simulink model "test_bu01_2018b_tuning"  (R2018b)
settings: Solver=FixedStepAuto  StartTime=0.0  StopTime=10  FixedStep=0.001  RelTol=1e-3
model workspace (MAT data in the model file):
  B1 = 0.0229925610147
  B2 = -0.371283802987
  B3 = -0.920624315565
  B4 = -0.0418343375444
  B5 = -0.493210333206
  B6 = 0
  B7 = -0.0892006103314
  B8 = -0.433620647544
  Ixx = 0.8
  Iyy = 2.075
  Izz = 1.25
  K = 0.92
  K1 = 0.96
  M1 = [1 1 -1 0.151123095698]
  M2 = [1 0 1 0.728919165533]
  M3 = [-1 0 -1 0]
  M4 = [-1 1 1 0.279370204784]
  M5 = [0 -1 0 0.953177368176]
  M6 = [0 -1 0 -1]
  M7 = [0 -1 0 0.164756597211]
  M8 = [0 -1 0 0.72330475505]
  Mass = 11.5
  b = 0
libraries: simulink x4, vrlib x4, shared6dof x1
(part 1 of 3)
settings Model: Creator=Administrator  LastModifiedBy=39926
settings DataIOCC: ReturnWorkspaceOutputs=on

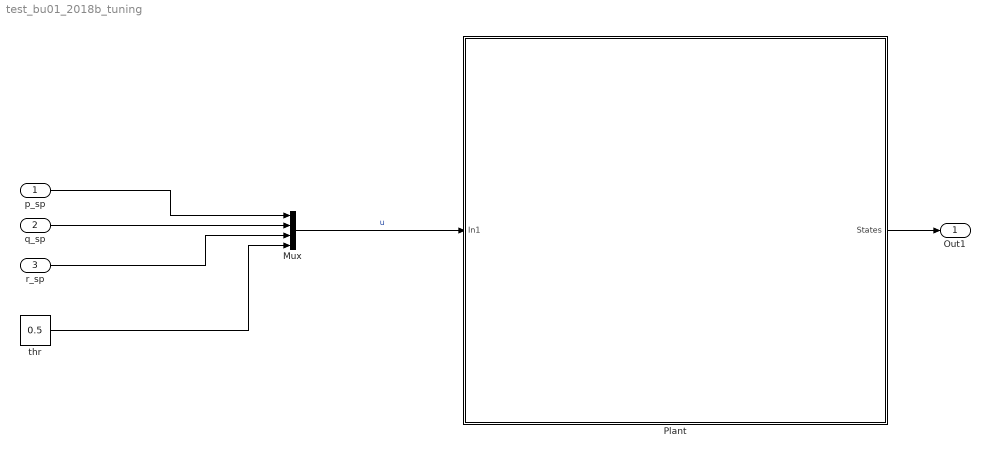
== system test_bu01_2018b_tuning ==
  "p_sp " : Inport
  q_sp : Inport  Port=2
  "r_sp " : Inport  Port=3
  Mux : Mux
  Plant : Subsystem
      mask Display: image('airframe.jpg');
  thr : Constant  Value=0.5
  Out1 : Outport
  wires:
  Mux/1 -> Plant/1(In1)  "u"
  q_sp/1 -> Mux/2
  "r_sp "/1 -> Mux/3
  Plant/1(States) -> Out1/1
  thr/1 -> Mux/4
  "p_sp "/1 -> Mux/1

== system test_bu01_2018b_tuning/Plant ==
  In1 : Inport
  Demux{,1..3} (4 alike) : Demux  Outputs=3
  Terminator{,3,5..9} (7 alike) : Terminator
  bu01_model : Subsystem  mask{Density=1.185}
      mask prompts: Density "空气密度D"
  混控器 : Subsystem
  Out Bus Element : Outport  PortName=States  Element=Xe
  Out Bus Element1 : Outport  PortName=States  Element=Ye
  Out Bus Element2 : Outport  PortName=States  Element=Ze
  Out Bus Element3 : Outport  PortName=States  Element=phi
  Out Bus Element4 : Outport  PortName=States  Element=theta
  Out Bus Element5 : Outport  PortName=States  Element=psi
  Out Bus Element6 : Outport  PortName=States  Element=u
  Out Bus Element7 : Outport  PortName=States  Element=v
  Out Bus Element8 : Outport  PortName=States  Element=w
  Out Bus Element9 : Outport  PortName=States  Element=p
  Out Bus Element10 : Outport  PortName=States  Element=q
  Out Bus Element11 : Outport  PortName=States  Element=r
  wires:
  混控器/1(PWM) -> bu01_model/1(PWM)
  bu01_model/6(Wb) -> Demux3/1
  bu01_model/7(dw/dt) -> Terminator5/1
  In1/1 -> 混控器/1(CtrlIn)
  bu01_model/1(Ve) -> Terminator/1
  bu01_model/3(ang) -> Demux1/1
  bu01_model/2(Xe) -> Demux/1
  bu01_model/4(DCM_e2b) -> Terminator3/1
  bu01_model/5(Vb) -> Demux2/1
  bu01_model/8(Abb) -> Terminator6/1
  bu01_model/9(T) -> Terminator7/1
  bu01_model/10(M) -> Terminator8/1
  bu01_model/11(Abe) -> Terminator9/1
  Demux/1 -> Out Bus Element/1
  Demux/2 -> Out Bus Element1/1
  Demux/3 -> Out Bus Element2/1
  Demux1/1 -> Out Bus Element3/1
  Demux1/2 -> Out Bus Element4/1
  Demux1/3 -> Out Bus Element5/1
  Demux2/1 -> Out Bus Element6/1
  Demux2/2 -> Out Bus Element7/1
  Demux2/3 -> Out Bus Element8/1
  Demux3/2 -> Out Bus Element10/1
  Demux3/1 -> Out Bus Element9/1
  Demux3/3 -> Out Bus Element11/1

== system test_bu01_2018b_tuning/Plant/bu01_model ==
  PWM : Inport
  6DOF (Quaternion) : shared6dof/6DOF (Euler Angles)  units=Metric (MKS)  mtype=Fixed  rep=Quaternion  xme_0=[0 0 0]  Vm_0=[0 0 0]  eul_0=[0 0 0]  pm_0=[0 0 0]  mass_0=Mass  mass_e=0.5  mass_f=2.0  inertia=[Ixx 0 0; 0 Iyy 0;0 0 Izz]  inertia_e=eye(3)  inertia_f=2*eye(3)  k_quat=1.0  vre_flag=on  abi_flag=on  aMode=0  xme_statename=''  Vm_statename=''  eul_statename=''  quat_statename=''  pm_statename=''  mass_statename=''
      settings: SourceProductBaseCode=AE
  Add : Sum  Inputs=3
  Add1 : Sum
  Constant : Constant  Value=Density
  Constant1 : Constant  Value=[0 0 0]
  Constant2 : Constant  Value=[0 0 0]
  PWM2Um : Subsystem
  动力系统模型 : Subsystem
  空气动力模型 : ModelReference  ModelNameDialog=BU01AM.slx  SimulationMode=Normal  ModelReferenceVersion=1.55
  重力模型 : Subsystem  mask{G=9.81, m=11.5}
      mask prompts: G "重力加速度G"; m "质量m"
  Ve : Outport
  Xe : Outport  Port=2
  ang : Outport  Port=3
  DCM_e2b : Outport  Port=4
  Vb : Outport  Port=5
  Wb : Outport  Port=6
  dw/dt : Outport  Port=7
  Abb : Outport  Port=8
  T : Outport  Port=9
  M : Outport  Port=10
  Abe : Outport  Port=11
  wires:
  Add1/1 -> M/1, 6DOF (Quaternion)/2  "M"
  6DOF (Quaternion)/1 -> Ve/1
  6DOF (Quaternion)/3 -> ang/1
  6DOF (Quaternion)/2 -> Xe/1
  6DOF (Quaternion)/4 -> 重力模型/1(DCM_e2b), DCM_e2b/1
  Add/1 -> T/1, 6DOF (Quaternion)/1  "T"
  6DOF (Quaternion)/7 -> dw/dt/1
  6DOF (Quaternion)/8 -> Abb/1
  6DOF (Quaternion)/5 -> Vb/1
  6DOF (Quaternion)/6 -> 空气动力模型/2, Wb/1
  6DOF (Quaternion)/9 -> Abe/1
  Constant/1 -> 空气动力模型/4
  重力模型/1(Fb_mg) -> Add/1  "mg_F"
  动力系统模型/1(Fb) -> Add/2  "Mot_F"
  空气动力模型/1 -> Add/3  "AM_F"
  空气动力模型/2 -> Add1/2  "AM_M"
  动力系统模型/2(Mb) -> Add1/1  "Mot_M"
  Constant1/1 -> 空气动力模型/3, 动力系统模型/3(Wb)
  Constant2/1 -> 空气动力模型/1, 动力系统模型/2(Vb)
  PWM/1 -> PWM2Um/1(PWM)
  PWM2Um/1(Um) -> 动力系统模型/1("Um ")

== system test_bu01_2018b_tuning/Plant/混控器 ==
  note: 机体构型描述：
      |           ^
      |           ||
      | 1P   -  ||  -   4N
      | 2N   -  ||  -   3P
      |            ||
      |            ||
      | -------------------
      | 5N  6N   7N 8N
  CtrlIn : Inport
  Bias{1..4} (4 alike) : Bias  Bias=[0 b 0 b]
  Demux : Demux  Outputs=8
  Gain : Gain  Gain="[1 1  -1 1]"
  Gain1 : Gain  Gain="[1 0  1 1]"
  Gain10 : Gain  Gain=K1
  Gain11 : Gain  Gain=K
  Gain2 : Gain  Gain=[-1 0 -1 1]
  Gain3 : Gain  Gain=[-1 1 1 1]
  Gain{4..6,8} (4 alike) : Gain  Gain=[0 -1 0 1]
  Gain7 : Gain  Gain=K
  Gain9 : Gain  Gain=K1
  Mux : Mux  Inputs=8
  Saturation : Saturate  UpperLimit=1  LowerLimit=0
  Scope : Scope
  Scope1 : Scope  NumInputPorts=8
  Sum of Elements{,1..7} (8 alike) : Sum  Inputs=+
  PWM : Outport
  wires:
  Sum of Elements/1 -> Mux/1
  Gain/1 -> Sum of Elements/1
  Gain2/1 -> Sum of Elements2/1
  Gain3/1 -> Sum of Elements3/1
  CtrlIn/1 -> Scope/1, Gain3/1, Gain4/1, Gain5/1, Gain8/1, Gain6/1, Gain1/1, Gain/1, Gain2/1
  Gain1/1 -> Sum of Elements1/1
  Bias3/1 -> Sum of Elements7/1
  Saturation/1 -> PWM/1, Demux/1
  Sum of Elements1/1 -> Mux/2
  Sum of Elements2/1 -> Mux/3
  Sum of Elements3/1 -> Mux/4
  Sum of Elements4/1 -> Mux/5
  Sum of Elements5/1 -> Mux/6
  Sum of Elements6/1 -> Mux/7
  Sum of Elements7/1 -> Mux/8
  Demux/1 -> Scope1/1  "m1"
  Demux/2 -> Scope1/2  "m2"
  Demux/3 -> Scope1/3  "m3"
  Demux/4 -> Scope1/4  "m4"
  Demux/5 -> Scope1/5  "m5"
  Demux/6 -> Scope1/6  "m6"
  Demux/7 -> Scope1/7  "m7"
  Demux/8 -> Scope1/8  "m8"
  Gain7/1 -> Bias3/1
  Gain8/1 -> Gain7/1
  Bias1/1 -> Sum of Elements6/1
  Gain6/1 -> Gain9/1
  Gain9/1 -> Bias1/1
  Bias2/1 -> Sum of Elements5/1
  Gain5/1 -> Gain10/1
  Gain10/1 -> Bias2/1
  Bias4/1 -> Sum of Elements4/1
  Gain4/1 -> Gain11/1
  Gain11/1 -> Bias4/1
  Mux/1 -> Saturation/1

== system test_bu01_2018b_tuning/Plant/bu01_model/PWM2Um ==
  PWM : Inport
  120AESC : Subsystem
  40AESC : Subsystem
  Constant2 : Constant  Value=25.2
  Demux : Demux  Outputs=2
  Demux1 : Demux  Outputs=8
  Mux : Mux  Inputs=2
  Saturation : Saturate  UpperLimit=1  LowerLimit=0
  Scope : Scope  NumInputPorts=8
  Um : Outport
  wires:
  Saturation/1 -> Demux/1
  PWM/1 -> Saturation/1
  120AESC/1(Out1) -> Mux/2
  Mux/1 -> Demux1/1, Um/1
  Demux1/1 -> Scope/1
  Demux1/2 -> Scope/2
  Demux1/3 -> Scope/3
  Demux1/4 -> Scope/4
  Demux1/5 -> Scope/5
  Demux1/6 -> Scope/6
  Demux1/7 -> Scope/7
  Demux1/8 -> Scope/8
  Constant2/1 -> 120AESC/2(Voltage_in), 40AESC/2(Votlage_in)
  Demux/1 -> 40AESC/1(Throttle_in)
  40AESC/1(Votlage_out) -> Mux/1
  Demux/2 -> 120AESC/1(Throttle_in)

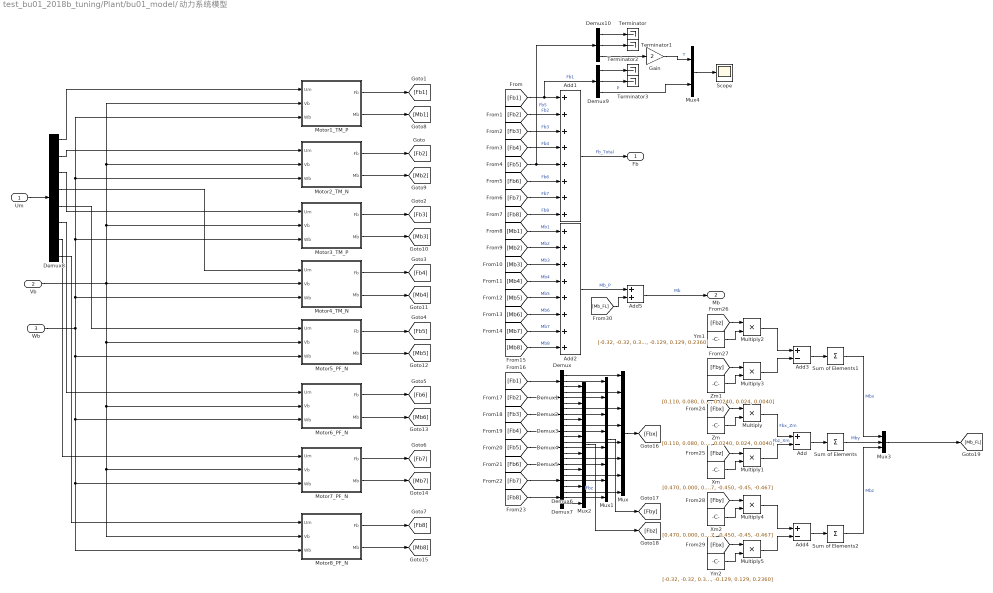
== system test_bu01_2018b_tuning/Plant/bu01_model/动力系统模型 ==
  "Um " : Inport
  Vb : Inport  Port=2
  Wb : Inport  Port=3
  Add : Sum  Inputs=+-
  Add1 : Sum  Inputs=8
  Add2 : Sum  Inputs=8
  Add3 : Sum  Inputs=+-
  Add4 : Sum  Inputs=+-
  Add5 : Sum
  Demux{,1..7,9..10} (10 alike) : Demux  Outputs=3
  Demux8 : Demux  Outputs=8
  Gain : Gain  Gain=2
  Motor1_TM_P : Subsystem
  Motor2_TM_N : Subsystem
  Motor3_TM_P : Subsystem
  Motor4_TM_N : Subsystem
  Motor5_PF_N : Subsystem
  Motor6_PF_N : Subsystem
  Motor7_PF_N : Subsystem
  Motor8_PF_N : Subsystem
  Multiply{,1..5} (6 alike) : Product
  Mux : Mux  Inputs=8
  Mux1 : Mux  Inputs=8
  Mux2 : Mux  Inputs=8
  Mux3 : Mux  Inputs=3
  Mux4 : Mux  Inputs=2
  Scope : Scope
  Sum of Elements : Sum  Inputs=+
  Sum of Elements1 : Sum  Inputs=+
  Sum of Elements2 : Sum  Inputs=+
  Terminator{,1..3} (4 alike) : Terminator
  Xm : Constant  Value=[0.470, 0.000, 0.00, 0.47, -0.467, -0.450, -0.45, -0.467]
  Xm2 : Constant  Value=[0.470, 0.000, 0.00, 0.47, -0.467, -0.450, -0.45, -0.467]
  Ym1 : Constant  Value=[-0.32, -0.32, 0.32, 0.32, -0.236, -0.129, 0.129, 0.2360]
  Ym2 : Constant  Value=[-0.32, -0.32, 0.32, 0.32, -0.236, -0.129, 0.129, 0.2360]
  Zm : Constant  Value=[0.110, 0.080, 0.08, 0.11, 0.0040, 0.0240, 0.024, 0.0040]
  Zm1 : Constant  Value=[0.110, 0.080, 0.08, 0.11, 0.0040, 0.0240, 0.024, 0.0040]
  Fb : Outport
  Mb : Outport  Port=2
  wires:
  Mux4/1 -> Scope/1
  Gain/1 -> Mux4/1  "T"
  Demux10/3 -> Gain/1
  Demux9/3 -> Mux4/2  "P"
  Demux9/2 -> Terminator3/1
  Demux9/1 -> Terminator2/1
  Demux10/2 -> Terminator1/1
  Demux10/1 -> Terminator/1
  Vb/1 -> Motor4_TM_N/2(Vb), Motor3_TM_P/2(Vb), Motor1_TM_P/2(Vb), Motor2_TM_N/2(Vb), Motor5_PF_N/2(Vb), Motor6_PF_N/2(Vb), Motor8_PF_N/2(Vb), Motor7_PF_N/2(Vb)
  Wb/1 -> Motor5_PF_N/3(Wb), Motor6_PF_N/3(Wb), Motor8_PF_N/3(Wb), Motor7_PF_N/3(Wb), Motor4_TM_N/3(Wb), Motor3_TM_P/3(Wb), Motor1_TM_P/3(Wb), Motor2_TM_N/3(Wb)
  Motor1_TM_P/1(Fb) -> [Fb1]
  Motor2_TM_N/1(Fb) -> [Fb2]
  Motor3_TM_P/1(Fb) -> [Fb3]
  Motor4_TM_N/1(Fb) -> [Fb4]
  Motor5_PF_N/1(Fb) -> [Fb5]
  Motor6_PF_N/1(Fb) -> [Fb6]
  Motor7_PF_N/1(Fb) -> [Fb7]
  Motor8_PF_N/1(Fb) -> [Fb8]
  Motor1_TM_P/2(Mb) -> [Mb1]
  Motor3_TM_P/2(Mb) -> [Mb3]
  Motor4_TM_N/2(Mb) -> [Mb4]
  Motor5_PF_N/2(Mb) -> [Mb5]
  Motor6_PF_N/2(Mb) -> [Mb6]
  Motor7_PF_N/2(Mb) -> [Mb7]
  Motor8_PF_N/2(Mb) -> [Mb8]
  [Fb8] -> Add1/8  "Fb8"
  [Fb7] -> Add1/7  "Fb7"
  [Fb6] -> Add1/6  "Fb6"
  [Fb5] -> Add1/5, Demux10/1  "Fb5"
  [Fb4] -> Add1/4  "Fb4"
  [Fb3] -> Add1/3  "Fb3"
  [Fb2] -> Add1/2  "Fb2"
  [Fb1] -> Add1/1, Demux9/1  "Fb1"
  Add1/1 -> Fb/1  "Fb_Total"
  [Mb1] -> Add2/1  "Mb1"
  [Mb4] -> Add2/4  "Mb4"
  [Mb3] -> Add2/3  "Mb3"
  [Mb2] -> Add2/2  "Mb2"
  [Mb5] -> Add2/5  "Mb5"
  [Mb6] -> Add2/6  "Mb6"
  [Mb7] -> Add2/7  "Mb7"
  [Mb8] -> Add2/8  "Mb8"
  [Fb1] -> Demux/1
  [Fb3] -> Demux2/1
  [Fb7] -> Demux6/1
  [Fb8] -> Demux7/1
  [Fb2] -> Demux1/1
  [Fb4] -> Demux3/1
  [Fb6] -> Demux5/1
  [Fb5] -> Demux4/1
  Demux/1 -> Mux/1
  Demux1/1 -> Mux/2
  Demux2/1 -> Mux/3
  Demux3/1 -> Mux/4
  Demux4/1 -> Mux/5
  Demux5/1 -> Mux/6
  Demux6/1 -> Mux/7
  Demux7/1 -> Mux/8
  Demux/2 -> Mux1/1
  Demux1/2 -> Mux1/2
  Demux2/2 -> Mux1/3
  Demux3/2 -> Mux1/4
  Demux4/2 -> Mux1/5
  Demux5/2 -> Mux1/6
  Demux6/2 -> Mux1/7
  Demux7/2 -> Mux1/8
  Demux/3 -> Mux2/1
  Demux1/3 -> Mux2/2
  Demux2/3 -> Mux2/3
  Demux3/3 -> Mux2/4
  Demux4/3 -> Mux2/5
  Demux5/3 -> Mux2/6
  Demux6/3 -> Mux2/7
  Demux7/3 -> Mux2/8
  Mux/1 -> [Fbx]
  Mux1/1 -> [Fby]
  Mux2/1 -> [Fbz]  "Fbz"
  [Fbx] -> Multiply/1
  Zm/1 -> Multiply/2
  Multiply/1 -> Add/1  "Fbx_Zm"
  [Fbz] -> Multiply1/1
  Xm/1 -> Multiply1/2
  Multiply1/1 -> Add/2  "Fbz_Xm"
  Add/1 -> Sum of Elements/1
  Sum of Elements/1 -> Mux3/2  "Mby"
  [Fbz] -> Multiply2/1
  Multiply2/1 -> Add3/1
  Zm1/1 -> Multiply3/2
  [Fby] -> Multiply3/1
  Ym1/1 -> Multiply2/2
  Sum of Elements1/1 -> Mux3/1  "Mbx"
  Add3/1 -> Sum of Elements1/1
  Multiply3/1 -> Add3/2
  [Fby] -> Multiply4/1
  Multiply4/1 -> Add4/1
  Ym2/1 -> Multiply5/2
  [Fbx] -> Multiply5/1
  Xm2/1 -> Multiply4/2
  Sum of Elements2/1 -> Mux3/3  "Mbz"
  Add4/1 -> Sum of Elements2/1
  Multiply5/1 -> Add4/2
  Mux3/1 -> [Mb_FL]
  [Mb_FL] -> Add5/2
  Add2/1 -> Add5/1  "Mb_P"
  Add5/1 -> Mb/1  "Mb"
  "Um "/1 -> Demux8/1
  Demux8/1 -> Motor1_TM_P/1(Um)
  Demux8/2 -> Motor2_TM_N/1(Um)
  Demux8/3 -> Motor3_TM_P/1(Um)
  Demux8/4 -> Motor4_TM_N/1(Um)
  Demux8/5 -> Motor5_PF_N/1(Um)
  Demux8/6 -> Motor6_PF_N/1(Um)
  Demux8/7 -> Motor7_PF_N/1(Um)
  Demux8/8 -> Motor8_PF_N/1(Um)
  Motor2_TM_N/2(Mb) -> [Mb2]

== system test_bu01_2018b_tuning/Plant/bu01_model/重力模型 ==
  DCM_e2b : Inport
  Constant : Constant  Value=[0 0 m*G]
  Multiply : Product  Multiplication=Matrix(*)
  Fb_mg : Outport
  wires:
  DCM_e2b/1 -> Multiply/1
  Constant/1 -> Multiply/2
  Multiply/1 -> Fb_mg/1

== system test_bu01_2018b_tuning/Plant/bu01_model/PWM2Um/120AESC ==
  Throttle_in : Inport  PortDimensions=4
  Voltage_in : Inport  Port=2
  Multiply 线性调节输出电压 : Product
  Saturation 限制油门最大最小值[0.0,1.0] : Saturate  UpperLimit=1.0  LowerLimit=0.0
  Transport Delay 模拟电调纯延时0.02秒 : TransportDelay  DelayTime=0.02
  Out1 : Outport
  wires:
  Multiply 线性调节输出电压/1 -> Out1/1  "Votlage_out"
  Voltage_in/1 -> Multiply 线性调节输出电压/2  "Voltage_in"
  Transport Delay 模拟电调纯延时0.02秒/1 -> Saturation 限制油门最大最小值[0.0,1.0]/1  "Throottle_dl"
  Throttle_in/1 -> Transport Delay 模拟电调纯延时0.02秒/1  "Throttle"
  Saturation 限制油门最大最小值[0.0,1.0]/1 -> Multiply 线性调节输出电压/1  "Throttle_ld"

== system test_bu01_2018b_tuning/Plant/bu01_model/PWM2Um/40AESC ==
  Throttle_in : Inport  PortDimensions=4
  Votlage_in : Inport  Port=2
  Constant 常数项 : Constant  Value=0.0629
  Constant1 一次项系数 : Constant  Value=0.9074
  Constant1 三次项系数2 : Constant  Value=-0.2904
  Constant1 二次项系数1 : Constant  Value=0.3398
  Constant1 幂级数 : Constant  Value=3
  Multiply{,1..3} (4 alike) : Product
  Plus : Sum  Inputs=++++
  Pow : Math  Operator=pow  RndMeth=Zero  SaturateOnIntegerOverflow=on
  Saturation 限制油门最大最小值[0.0,1.0] : Saturate  UpperLimit=1.0  LowerLimit=0.0
  Square : Math  Operator=square  SaturateOnIntegerOverflow=on
  Transport Delay 模拟电调纯延时0.02秒 : TransportDelay  DelayTime=0.02
  Votlage_out : Outport
  wires:
  Multiply1/1 -> Votlage_out/1
  Votlage_in/1 -> Multiply1/2
  Saturation 限制油门最大最小值[0.0,1.0]/1 -> Pow/1, Square/1, Multiply/1  "Throttle_ld"
  Transport Delay 模拟电调纯延时0.02秒/1 -> Saturation 限制油门最大最小值[0.0,1.0]/1  "Throttle_dl"
  Constant1 一次项系数/1 -> Multiply/2
  Constant 常数项/1 -> Plus/1
  Multiply/1 -> Plus/2
  Multiply2/1 -> Plus/3
  Throttle_in/1 -> Transport Delay 模拟电调纯延时0.02秒/1
  Constant1 三次项系数2/1 -> Multiply3/2
  Constant1 二次项系数1/1 -> Multiply2/2
  Constant1 幂级数/1 -> Pow/2
  Square/1 -> Multiply2/1
  Pow/1 -> Multiply3/1
  Plus/1 -> Multiply1/1  "Throttle_out"
  Multiply3/1 -> Plus/4

== system test_bu01_2018b_tuning/Plant/bu01_model/动力系统模型/Motor1_TM_P ==
  Um : Inport
  Vb : Inport  Port=2
  Wb : Inport  Port=3
  Constant : Constant  Value=[0 0 -1]
  Constant1 : Constant  Value=1.185
  Gain : Gain  Gain=1/60
  "TM1654P " : Subsystem
  "TMU5KV400 " : Subsystem
  Terminator : Terminator
  Fb : Outport
  Mb : Outport  Port=2
  wires:
  Constant1/1 -> "TM1654P "/4(Density)
  Wb/1 -> "TM1654P "/2(Wb)
  Vb/1 -> "TM1654P "/1(Vb)
  Constant/1 -> "TM1654P "/3(Ax)
  "TMU5KV400 "/1(Im) -> Terminator/1
  Gain/1 -> "TM1654P "/5(Ns)
  "TMU5KV400 "/2(RPM) -> Gain/1
  "TM1654P "/2(Mb) -> Mb/1  "Mb"
  "TM1654P "/1(Fb) -> Fb/1  "Fb"
  "TM1654P "/3(Tq) -> "TMU5KV400 "/2(Tq)
  "TM1654P "/4(Izz) -> "TMU5KV400 "/3(Izz)
  Um/1 -> "TMU5KV400 "/1(Um)

== system test_bu01_2018b_tuning/Plant/bu01_model/动力系统模型/Motor2_TM_N ==
  Um : Inport
  Vb : Inport  Port=2
  Wb : Inport  Port=3
  Constant2 : Constant  Value=[0 0 -1]
  Constant3 : Constant  Value=1.185
  Gain1 : Gain  Gain=1/60
  "TM1654N " : Subsystem
  "TMU5KV400 " : Subsystem
  Terminator1 : Terminator
  Fb : Outport
  Mb : Outport  Port=2
  wires:
  Constant2/1 -> "TM1654N "/3(Ax)
  "TM1654N "/4(Izz) -> "TMU5KV400 "/3(Izz)
  "TM1654N "/1(Fb) -> Fb/1  "Fb"
  "TMU5KV400 "/1(Im) -> Terminator1/1
  Constant3/1 -> "TM1654N "/4(Density)
  "TM1654N "/3(Tq) -> "TMU5KV400 "/2(Tq)
  Wb/1 -> "TM1654N "/2(Wb)
  Gain1/1 -> "TM1654N "/5(Ns)
  Um/1 -> "TMU5KV400 "/1(Um)
  "TM1654N "/2(Mb) -> Mb/1  "Mb"
  "TMU5KV400 "/2(RPM) -> Gain1/1
  Vb/1 -> "TM1654N "/1(Vb)

== system test_bu01_2018b_tuning/Plant/bu01_model/动力系统模型/Motor3_TM_P ==
  Um : Inport
  Vb : Inport  Port=2
  Wb : Inport  Port=3
  Constant : Constant  Value=[0 0 -1]
  Constant1 : Constant  Value=1.185
  Gain : Gain  Gain=1/60
  "TM1654P " : Subsystem
  "TMU5KV400 " : Subsystem
  Terminator : Terminator
  Fb : Outport
  Mb : Outport  Port=2
  wires:
  Constant1/1 -> "TM1654P "/4(Density)
  Wb/1 -> "TM1654P "/2(Wb)
  Vb/1 -> "TM1654P "/1(Vb)
  Constant/1 -> "TM1654P "/3(Ax)
  "TMU5KV400 "/1(Im) -> Terminator/1
  Gain/1 -> "TM1654P "/5(Ns)
  "TMU5KV400 "/2(RPM) -> Gain/1
  "TM1654P "/2(Mb) -> Mb/1  "Mb"
  "TM1654P "/1(Fb) -> Fb/1  "Fb"
  "TM1654P "/3(Tq) -> "TMU5KV400 "/2(Tq)
  "TM1654P "/4(Izz) -> "TMU5KV400 "/3(Izz)
  Um/1 -> "TMU5KV400 "/1(Um)

== system test_bu01_2018b_tuning/Plant/bu01_model/动力系统模型/Motor4_TM_N ==
  Um : Inport
  Vb : Inport  Port=2
  Wb : Inport  Port=3
  Constant : Constant  Value=[0 0 -1]
  Constant3 : Constant  Value=1.185
  Gain1 : Gain  Gain=1/60
  "TM1654N " : Subsystem
  "TMU5KV400 " : Subsystem
  Terminator1 : Terminator
  Fb : Outport
  Mb : Outport  Port=2
  wires:
  Constant/1 -> "TM1654N "/3(Ax)
  "TM1654N "/4(Izz) -> "TMU5KV400 "/3(Izz)
  "TM1654N "/1(Fb) -> Fb/1  "Fb"
  "TMU5KV400 "/1(Im) -> Terminator1/1
  Constant3/1 -> "TM1654N "/4(Density)
  "TM1654N "/3(Tq) -> "TMU5KV400 "/2(Tq)
  Wb/1 -> "TM1654N "/2(Wb)
  Gain1/1 -> "TM1654N "/5(Ns)
  Um/1 -> "TMU5KV400 "/1(Um)
  "TM1654N "/2(Mb) -> Mb/1  "Mb"
  "TMU5KV400 "/2(RPM) -> Gain1/1
  Vb/1 -> "TM1654N "/1(Vb)

== system test_bu01_2018b_tuning/Plant/bu01_model/动力系统模型/Motor5_PF_N ==
  Um : Inport
  Vb : Inport  Port=2
  Wb : Inport  Port=3
  Constant : Constant  Value=[0 0 -1]
  Constant1 : Constant  Value=1.185
  Gain : Gain  Gain=1/60
  PF70mmDuctFanN : Subsystem
  PFKV2300 : Subsystem
  Terminator : Terminator
  Fb : Outport
  Mb : Outport  Port=2
  wires:
  Um/1 -> PFKV2300/1(Um)
  PF70mmDuctFanN/4(Izz) -> PFKV2300/3(Izz)
  PF70mmDuctFanN/3(Tq) -> PFKV2300/2(Tq)
  PF70mmDuctFanN/1(Fb) -> Fb/1  "Fb"
  PF70mmDuctFanN/2(Mb) -> Mb/1  "Mb"
  PFKV2300/2(RPM) -> Gain/1
  PFKV2300/1(Im) -> Terminator/1
  Constant/1 -> PF70mmDuctFanN/3(Ax_ip)
  Vb/1 -> PF70mmDuctFanN/1(Vb_ip)
  Wb/1 -> PF70mmDuctFanN/2(Wb_ip)
  Gain/1 -> PF70mmDuctFanN/4(Ns_ip)
  Constant1/1 -> PF70mmDuctFanN/5(Pro)

== system test_bu01_2018b_tuning/Plant/bu01_model/动力系统模型/Motor6_PF_N ==
  Um : Inport
  Vb : Inport  Port=2
  Wb : Inport  Port=3
  Constant : Constant  Value=[0 0 -1]
  Constant1 : Constant  Value=1.185
  Gain : Gain  Gain=1/60
  PF70mmDuctFanN : Subsystem
  PFKV2300 : Subsystem
  Terminator : Terminator
  Fb : Outport
  Mb : Outport  Port=2
  wires:
  Um/1 -> PFKV2300/1(Um)
  PF70mmDuctFanN/4(Izz) -> PFKV2300/3(Izz)
  PF70mmDuctFanN/3(Tq) -> PFKV2300/2(Tq)
  PF70mmDuctFanN/1(Fb) -> Fb/1  "Fb"
  PF70mmDuctFanN/2(Mb) -> Mb/1  "Mb"
  PFKV2300/2(RPM) -> Gain/1
  PFKV2300/1(Im) -> Terminator/1
  Constant/1 -> PF70mmDuctFanN/3(Ax_ip)
  Vb/1 -> PF70mmDuctFanN/1(Vb_ip)
  Wb/1 -> PF70mmDuctFanN/2(Wb_ip)
  Gain/1 -> PF70mmDuctFanN/4(Ns_ip)
  Constant1/1 -> PF70mmDuctFanN/5(Pro)

== system test_bu01_2018b_tuning/Plant/bu01_model/动力系统模型/Motor7_PF_N ==
  Um : Inport
  Vb : Inport  Port=2
  Wb : Inport  Port=3
  Constant : Constant  Value=[0 0 -1]
  Constant1 : Constant  Value=1.185
  Gain : Gain  Gain=1/60
  PF70mmDuctFanN : Subsystem
  PFKV2300 : Subsystem
  Terminator : Terminator
  Fb : Outport
  Mb : Outport  Port=2
  wires:
  Um/1 -> PFKV2300/1(Um)
  PF70mmDuctFanN/4(Izz) -> PFKV2300/3(Izz)
  PF70mmDuctFanN/3(Tq) -> PFKV2300/2(Tq)
  PF70mmDuctFanN/1(Fb) -> Fb/1  "Fb"
  PF70mmDuctFanN/2(Mb) -> Mb/1  "Mb"
  PFKV2300/2(RPM) -> Gain/1
  PFKV2300/1(Im) -> Terminator/1
  Constant/1 -> PF70mmDuctFanN/3(Ax_ip)
  Vb/1 -> PF70mmDuctFanN/1(Vb_ip)
  Wb/1 -> PF70mmDuctFanN/2(Wb_ip)
  Gain/1 -> PF70mmDuctFanN/4(Ns_ip)
  Constant1/1 -> PF70mmDuctFanN/5(Pro)

== system test_bu01_2018b_tuning/Plant/bu01_model/动力系统模型/Motor8_PF_N ==
  Um : Inport
  Vb : Inport  Port=2
  Wb : Inport  Port=3
  Constant : Constant  Value=[0 0 -1]
  Constant1 : Constant  Value=1.185
  Gain : Gain  Gain=1/60
  PF70mmDuctFanN : Subsystem
  PFKV2300 : Subsystem
  Terminator : Terminator
  Fb : Outport
  Mb : Outport  Port=2
  wires:
  Constant1/1 -> PF70mmDuctFanN/5(Pro)
  Gain/1 -> PF70mmDuctFanN/4(Ns_ip)
  Wb/1 -> PF70mmDuctFanN/2(Wb_ip)
  Vb/1 -> PF70mmDuctFanN/1(Vb_ip)
  Constant/1 -> PF70mmDuctFanN/3(Ax_ip)
  PFKV2300/1(Im) -> Terminator/1
  PFKV2300/2(RPM) -> Gain/1
  PF70mmDuctFanN/2(Mb) -> Mb/1  "Mb"
  PF70mmDuctFanN/1(Fb) -> Fb/1  "Fb"
  PF70mmDuctFanN/3(Tq) -> PFKV2300/2(Tq)
  PF70mmDuctFanN/4(Izz) -> PFKV2300/3(Izz)
  Um/1 -> PFKV2300/1(Um)

== system test_bu01_2018b_tuning/Plant/bu01_model/动力系统模型/Motor1_TM_P/TM1654P  ==
  Vb : Inport  PortDimensions=3
  Wb : Inport  Port=2  PortDimensions=3
  Ax : Inport  Port=3  PortDimensions=3
  Density : Inport  Port=4  PortDimensions=1
  Ns : Inport  Port=5  PortDimensions=1
  Bus Selector : BusSelector  OutputSignals=FM,Tq,Izz
  Bus Selector1 : BusSelector  OutputSignals=Fb,Mb
  Bus Creator : BusCreator  Inputs=5
  螺旋桨模型 : Subsystem  mask{Izz=0.00024, D=0.406, Fratio=1.125, Mratio=0.975}
      mask prompts: Izz "螺旋桨惯量Izz"; D "螺旋桨直径D"; Fratio "推力系数Fratio"; Mratio "力矩系数Mratio"
      mask Display: disp('螺旋桨模型')
  Fb : Outport
  Mb : Outport  Port=2
  Tq : Outport  Port=3
  Izz : Outport  Port=4
  wires:
  Bus Selector/1 -> Bus Selector1/1  "<FM>"
  Bus Selector/3 -> Izz/1  "<Izz>"
  Bus Selector1/2 -> Mb/1  "<Mb>"
  Wb/1 -> Bus Creator/2  "Wb"
  Bus Selector1/1 -> Fb/1  "<Fb>"
  Ax/1 -> Bus Creator/3  "Ax"
  Density/1 -> Bus Creator/4  "Density"
  Bus Selector/2 -> Tq/1  "<Tq>"
  螺旋桨模型/1(TM_OUT) -> Bus Selector/1
  Vb/1 -> Bus Creator/1  "Vb"
  Ns/1 -> Bus Creator/5  "Ns"
  Bus Creator/1 -> 螺旋桨模型/1(In1)

== system test_bu01_2018b_tuning/Plant/bu01_model/动力系统模型/Motor1_TM_P/TMU5KV400  ==
  Um : Inport  PortDimensions=1
  Tq : Inport  Port=2  PortDimensions=1
  Izz : Inport  Port=3  PortDimensions=1
  Bus Selector : BusSelector  OutputSignals=Im,RPM
  Bus Creator : BusCreator  Inputs=3
  DCMotor : Subsystem  mask{L=0.0000702, Km=0.026228988, Kemf=0.029486916, Imzz=0.00002, Ra=0.0993, I0=0.436382879}
      mask prompts: L "电感值L"; Km "转矩常量Km"; Kemf "反电动势Kemf"; Imzz "转子惯量Imzz"; Ra "电动机内阻Ra"; I0 "空载电流I0"
      mask Display: disp('DCMotor')
  Im : Outport
  RPM : Outport  Port=2
  wires:
  Bus Selector/2 -> RPM/1  "<RPM>"
  Bus Selector/1 -> Im/1  "<Im>"
  DCMotor/1(Out1) -> Bus Selector/1
  Um/1 -> Bus Creator/1  "Um"
  Bus Creator/1 -> DCMotor/1(In1)
  Izz/1 -> Bus Creator/3  "Izz"
  Tq/1 -> Bus Creator/2  "Tq"

== system test_bu01_2018b_tuning/Plant/bu01_model/动力系统模型/Motor2_TM_N/TM1654N  ==
  Vb : Inport  PortDimensions=3
  Wb : Inport  Port=2  PortDimensions=3
  Ax : Inport  Port=3  PortDimensions=3
  Density : Inport  Port=4  PortDimensions=1
  Ns : Inport  Port=5  PortDimensions=1
  Bus Selector : BusSelector  OutputSignals=FM,Tq,Izz
  Bus Selector1 : BusSelector  OutputSignals=Fb,Mb
  Bus Creator : BusCreator  Inputs=5
  螺旋桨模型 : Subsystem  mask{Izz=0.00024, D=0.406, Fratio=1.125, Mratio=0.975}
      mask prompts: Izz "螺旋桨惯量Izz"; D "螺旋桨直径D"; Fratio "推力系数Fratio"; Mratio "力矩系数Mratio"
      mask Display: disp('螺旋桨模型')
  Fb : Outport
  Mb : Outport  Port=2
  Tq : Outport  Port=3
  Izz : Outport  Port=4
  wires:
  Bus Selector/2 -> Tq/1  "<Tq>"
  Bus Selector1/1 -> Fb/1  "<Fb>"
  Bus Selector/1 -> Bus Selector1/1  "<FM>"
  Bus Selector/3 -> Izz/1  "<Izz>"
  Bus Selector1/2 -> Mb/1  "<Mb>"
  螺旋桨模型/1(TM_OUT) -> Bus Selector/1
  Vb/1 -> Bus Creator/1  "Vb"
  Bus Creator/1 -> 螺旋桨模型/1(In1)
  Wb/1 -> Bus Creator/2  "Wb"
  Ns/1 -> Bus Creator/5  "Ns"
  Ax/1 -> Bus Creator/3  "Ax"
  Density/1 -> Bus Creator/4  "Density"

== system test_bu01_2018b_tuning/Plant/bu01_model/动力系统模型/Motor2_TM_N/TMU5KV400  ==
  Um : Inport  PortDimensions=1
  Tq : Inport  Port=2  PortDimensions=1
  Izz : Inport  Port=3  PortDimensions=1
  Bus Selector : BusSelector  OutputSignals=Im,RPM
  Bus Creator : BusCreator  Inputs=3
  DCMotor1 : Subsystem  mask{L=0.0000702, Km=0.026228988, Kemf=0.029486916, Imzz=0.00002, Ra=0.0993, I0=0.436382879}
      mask prompts: L "电感值L"; Km "转矩常量Km"; Kemf "反电动势Kemf"; Imzz "转子惯量Imzz"; Ra "电动机内阻Ra"; I0 "空载电流I0"
      mask Display: disp('DCMotor')
  Im : Outport
  RPM : Outport  Port=2
  wires:
  Bus Selector/2 -> RPM/1  "<RPM>"
  Bus Selector/1 -> Im/1  "<Im>"
  DCMotor1/1(Out1) -> Bus Selector/1
  Um/1 -> Bus Creator/1  "Um"
  Bus Creator/1 -> DCMotor1/1(In1)
  Izz/1 -> Bus Creator/3  "Izz"
  Tq/1 -> Bus Creator/2  "Tq"

== system test_bu01_2018b_tuning/Plant/bu01_model/动力系统模型/Motor3_TM_P/TM1654P  ==
  Vb : Inport  PortDimensions=3
  Wb : Inport  Port=2  PortDimensions=3
  Ax : Inport  Port=3  PortDimensions=3
  Density : Inport  Port=4  PortDimensions=1
  Ns : Inport  Port=5  PortDimensions=1
  Bus Selector : BusSelector  OutputSignals=FM,Tq,Izz
  Bus Selector1 : BusSelector  OutputSignals=Fb,Mb
  Bus Creator : BusCreator  Inputs=5
  螺旋桨模型 : Subsystem  mask{Izz=0.00024, D=0.406, Fratio=1.125, Mratio=0.975}
      mask prompts: Izz "螺旋桨惯量Izz"; D "螺旋桨直径D"; Fratio "推力系数Fratio"; Mratio "力矩系数Mratio"
      mask Display: disp('螺旋桨模型')
  Fb : Outport
  Mb : Outport  Port=2
  Tq : Outport  Port=3
  Izz : Outport  Port=4
  wires:
  Bus Selector/1 -> Bus Selector1/1  "<FM>"
  Bus Selector/3 -> Izz/1  "<Izz>"
  Bus Selector1/2 -> Mb/1  "<Mb>"
  Wb/1 -> Bus Creator/2  "Wb"
  Bus Selector1/1 -> Fb/1  "<Fb>"
  Ax/1 -> Bus Creator/3  "Ax"
  Density/1 -> Bus Creator/4  "Density"
  Bus Selector/2 -> Tq/1  "<Tq>"
  螺旋桨模型/1(TM_OUT) -> Bus Selector/1
  Vb/1 -> Bus Creator/1  "Vb"
  Ns/1 -> Bus Creator/5  "Ns"
  Bus Creator/1 -> 螺旋桨模型/1(In1)

== system test_bu01_2018b_tuning/Plant/bu01_model/动力系统模型/Motor3_TM_P/TMU5KV400  ==
  Um : Inport  PortDimensions=1
  Tq : Inport  Port=2  PortDimensions=1
  Izz : Inport  Port=3  PortDimensions=1
  Bus Selector : BusSelector  OutputSignals=Im,RPM
  Bus Creator : BusCreator  Inputs=3
  DCMotor : Subsystem  mask{L=0.0000702, Km=0.026228988, Kemf=0.029486916, Imzz=0.00002, Ra=0.0993, I0=0.436382879}
      mask prompts: L "电感值L"; Km "转矩常量Km"; Kemf "反电动势Kemf"; Imzz "转子惯量Imzz"; Ra "电动机内阻Ra"; I0 "空载电流I0"
      mask Display: disp('DCMotor')
  Im : Outport
  RPM : Outport  Port=2
  wires:
  Bus Selector/2 -> RPM/1  "<RPM>"
  Bus Selector/1 -> Im/1  "<Im>"
  DCMotor/1(Out1) -> Bus Selector/1
  Um/1 -> Bus Creator/1  "Um"
  Bus Creator/1 -> DCMotor/1(In1)
  Izz/1 -> Bus Creator/3  "Izz"
  Tq/1 -> Bus Creator/2  "Tq"

== system test_bu01_2018b_tuning/Plant/bu01_model/动力系统模型/Motor4_TM_N/TM1654N  ==
  Vb : Inport  PortDimensions=3
  Wb : Inport  Port=2  PortDimensions=3
  Ax : Inport  Port=3  PortDimensions=3
  Density : Inport  Port=4  PortDimensions=1
  Ns : Inport  Port=5  PortDimensions=1
  Bus Selector : BusSelector  OutputSignals=FM,Tq,Izz
  Bus Selector1 : BusSelector  OutputSignals=Fb,Mb
  Bus Creator : BusCreator  Inputs=5
  螺旋桨模型 : Subsystem  mask{Izz=0.00024, D=0.406, Fratio=1.125, Mratio=0.975}
      mask prompts: Izz "螺旋桨惯量Izz"; D "螺旋桨直径D"; Fratio "推力系数Fratio"; Mratio "力矩系数Mratio"
      mask Display: disp('螺旋桨模型')
  Fb : Outport
  Mb : Outport  Port=2
  Tq : Outport  Port=3
  Izz : Outport  Port=4
  wires:
  Bus Selector/2 -> Tq/1  "<Tq>"
  Bus Selector1/1 -> Fb/1  "<Fb>"
  Bus Selector/1 -> Bus Selector1/1  "<FM>"
  Bus Selector/3 -> Izz/1  "<Izz>"
  Bus Selector1/2 -> Mb/1  "<Mb>"
  螺旋桨模型/1(TM_OUT) -> Bus Selector/1
  Vb/1 -> Bus Creator/1  "Vb"
  Bus Creator/1 -> 螺旋桨模型/1(In1)
  Wb/1 -> Bus Creator/2  "Wb"
  Ns/1 -> Bus Creator/5  "Ns"
  Ax/1 -> Bus Creator/3  "Ax"
  Density/1 -> Bus Creator/4  "Density"

== system test_bu01_2018b_tuning/Plant/bu01_model/动力系统模型/Motor4_TM_N/TMU5KV400  ==
  Um : Inport  PortDimensions=1
  Tq : Inport  Port=2  PortDimensions=1
  Izz : Inport  Port=3  PortDimensions=1
  Bus Selector : BusSelector  OutputSignals=Im,RPM
  Bus Creator : BusCreator  Inputs=3
  DCMotor1 : Subsystem  mask{L=0.0000702, Km=0.026228988, Kemf=0.029486916, Imzz=0.00002, Ra=0.0993, I0=0.436382879}
      mask prompts: L "电感值L"; Km "转矩常量Km"; Kemf "反电动势Kemf"; Imzz "转子惯量Imzz"; Ra "电动机内阻Ra"; I0 "空载电流I0"
      mask Display: disp('DCMotor')
  Im : Outport
  RPM : Outport  Port=2
  wires:
  Bus Selector/2 -> RPM/1  "<RPM>"
  Bus Selector/1 -> Im/1  "<Im>"
  DCMotor1/1(Out1) -> Bus Selector/1
  Um/1 -> Bus Creator/1  "Um"
  Bus Creator/1 -> DCMotor1/1(In1)
  Izz/1 -> Bus Creator/3  "Izz"
  Tq/1 -> Bus Creator/2  "Tq"

== system test_bu01_2018b_tuning/Plant/bu01_model/动力系统模型/Motor5_PF_N/PF70mmDuctFanN ==
  Vb_ip : Inport  PortDimensions=3
  Wb_ip : Inport  Port=2  PortDimensions=3
  Ax_ip : Inport  Port=3  PortDimensions=3
  Ns_ip : Inport  Port=4  PortDimensions=1
  Pro : Inport  Port=5  PortDimensions=1
  Bus Selector : BusSelector  OutputSignals=Fb&Mb,Tq,Izz
  Bus Selector1 : BusSelector  OutputSignals=Fb,Mb
  Bus Creator : BusCreator  Inputs=5
  "涵道风扇模型 " : Subsystem  mask{Fratio=1.125, Mratio=0.975, Tqratio=0.4, Izz=0.00000309}
      mask prompts: Fratio "涵道风扇气动力修正系数"; Mratio "涵道风扇气动力矩修正系数"; Tqratio "涵道风扇扭矩修正系数"; Izz "涵道风扇转动惯量"
  Fb : Outport
  Mb : Outport  Port=2
  Tq : Outport  Port=3
  Izz : Outport  Port=4
  wires:
  Pro/1 -> Bus Creator/5  "Pro"
  Bus Selector/2 -> Tq/1  "<Tq>"
  Bus Selector/3 -> Izz/1  "<Izz>"
  Bus Selector1/1 -> Fb/1  "<Fb>"
  Ns_ip/1 -> Bus Creator/4  "Ns"
  Bus Selector1/2 -> Mb/1  "<Mb>"
  Bus Selector/1 -> Bus Selector1/1  "<Fb&Mb>"
  Wb_ip/1 -> Bus Creator/2  "Wb"
  Bus Creator/1 -> "涵道风扇模型 "/1(In1)
  "涵道风扇模型 "/1(Out1) -> Bus Selector/1
  Ax_ip/1 -> Bus Creator/3  "Ax"
  Vb_ip/1 -> Bus Creator/1  "Vb"

== system test_bu01_2018b_tuning/Plant/bu01_model/动力系统模型/Motor5_PF_N/PFKV2300 ==
  Um : Inport  PortDimensions=1
  Tq : Inport  Port=2  PortDimensions=1
  Izz : Inport  Port=3  PortDimensions=1
  Bus Selector : BusSelector  OutputSignals=Im,RPM
  Bus Creator : BusCreator  Inputs=3
  DCMotor : Subsystem  mask{L=0.0053, Km=0.0041, Kemf=0.0041, Imzz=1e-05, Ra=0.045, I0=2.35}
      mask prompts: L "电感值L"; Km "转矩常量Km"; Kemf "反电动势Kemf"; Imzz "转子惯量Imzz"; Ra "电动机内阻Ra"; I0 "空载电流I0"
      mask Display: disp('DCMotor')
  Im : Outport
  RPM : Outport  Port=2
  wires:
  Bus Creator/1 -> DCMotor/1(In1)
  Um/1 -> Bus Creator/1  "Um"
  Izz/1 -> Bus Creator/3  "Izz"
  Bus Selector/2 -> RPM/1  "<RPM>"
  Tq/1 -> Bus Creator/2  "Tq"
  DCMotor/1(Out1) -> Bus Selector/1
  Bus Selector/1 -> Im/1  "<Im>"

== system test_bu01_2018b_tuning/Plant/bu01_model/动力系统模型/Motor6_PF_N/PF70mmDuctFanN ==
  Vb_ip : Inport  PortDimensions=3
  Wb_ip : Inport  Port=2  PortDimensions=3
  Ax_ip : Inport  Port=3  PortDimensions=3
  Ns_ip : Inport  Port=4  PortDimensions=1
  Pro : Inport  Port=5  PortDimensions=1
  Bus Selector : BusSelector  OutputSignals=Fb&Mb,Tq,Izz
  Bus Selector1 : BusSelector  OutputSignals=Fb,Mb
  Bus Creator : BusCreator  Inputs=5
  "涵道风扇模型 " : Subsystem  mask{Fratio=1.125, Mratio=0.975, Tqratio=0.4, Izz=0.00000309}
      mask prompts: Fratio "涵道风扇气动力修正系数"; Mratio "涵道风扇气动力矩修正系数"; Tqratio "涵道风扇扭矩修正系数"; Izz "涵道风扇转动惯量"
  Fb : Outport
  Mb : Outport  Port=2
  Tq : Outport  Port=3
  Izz : Outport  Port=4
  wires:
  Pro/1 -> Bus Creator/5  "Pro"
  Bus Selector/2 -> Tq/1  "<Tq>"
  Bus Selector/3 -> Izz/1  "<Izz>"
  Bus Selector1/1 -> Fb/1  "<Fb>"
  Ns_ip/1 -> Bus Creator/4  "Ns"
  Bus Selector1/2 -> Mb/1  "<Mb>"
  Bus Selector/1 -> Bus Selector1/1  "<Fb&Mb>"
  Wb_ip/1 -> Bus Creator/2  "Wb"
  Bus Creator/1 -> "涵道风扇模型 "/1(In1)
  "涵道风扇模型 "/1(Out1) -> Bus Selector/1
  Ax_ip/1 -> Bus Creator/3  "Ax"
  Vb_ip/1 -> Bus Creator/1  "Vb"

== system test_bu01_2018b_tuning/Plant/bu01_model/动力系统模型/Motor6_PF_N/PFKV2300 ==
  Um : Inport  PortDimensions=1
  Tq : Inport  Port=2  PortDimensions=1
  Izz : Inport  Port=3  PortDimensions=1
  Bus Selector : BusSelector  OutputSignals=Im,RPM
  Bus Creator : BusCreator  Inputs=3
  DCMotor : Subsystem  mask{L=0.0053, Km=0.0041, Kemf=0.0041, Imzz=1e-05, Ra=0.045, I0=2.35}
      mask prompts: L "电感值L"; Km "转矩常量Km"; Kemf "反电动势Kemf"; Imzz "转子惯量Imzz"; Ra "电动机内阻Ra"; I0 "空载电流I0"
      mask Display: disp('DCMotor')
  Im : Outport
  RPM : Outport  Port=2
  wires:
  Bus Creator/1 -> DCMotor/1(In1)
  Um/1 -> Bus Creator/1  "Um"
  Izz/1 -> Bus Creator/3  "Izz"
  Bus Selector/2 -> RPM/1  "<RPM>"
  Tq/1 -> Bus Creator/2  "Tq"
  DCMotor/1(Out1) -> Bus Selector/1
  Bus Selector/1 -> Im/1  "<Im>"

== system test_bu01_2018b_tuning/Plant/bu01_model/动力系统模型/Motor7_PF_N/PF70mmDuctFanN ==
  Vb_ip : Inport  PortDimensions=3
  Wb_ip : Inport  Port=2  PortDimensions=3
  Ax_ip : Inport  Port=3  PortDimensions=3
  Ns_ip : Inport  Port=4  PortDimensions=1
  Pro : Inport  Port=5  PortDimensions=1
  Bus Selector : BusSelector  OutputSignals=Fb&Mb,Tq,Izz
  Bus Selector1 : BusSelector  OutputSignals=Fb,Mb
  Bus Creator : BusCreator  Inputs=5
  "涵道风扇模型 " : Subsystem  mask{Fratio=1.125, Mratio=0.975, Tqratio=0.4, Izz=0.00000309}
      mask prompts: Fratio "涵道风扇气动力修正系数"; Mratio "涵道风扇气动力矩修正系数"; Tqratio "涵道风扇扭矩修正系数"; Izz "涵道风扇转动惯量"
  Fb : Outport
  Mb : Outport  Port=2
  Tq : Outport  Port=3
  Izz : Outport  Port=4
  wires:
  Pro/1 -> Bus Creator/5  "Pro"
  Bus Selector/2 -> Tq/1  "<Tq>"
  Bus Selector/3 -> Izz/1  "<Izz>"
  Bus Selector1/1 -> Fb/1  "<Fb>"
  Ns_ip/1 -> Bus Creator/4  "Ns"
  Bus Selector1/2 -> Mb/1  "<Mb>"
  Bus Selector/1 -> Bus Selector1/1  "<Fb&Mb>"
  Wb_ip/1 -> Bus Creator/2  "Wb"
  Bus Creator/1 -> "涵道风扇模型 "/1(In1)
  "涵道风扇模型 "/1(Out1) -> Bus Selector/1
  Ax_ip/1 -> Bus Creator/3  "Ax"
  Vb_ip/1 -> Bus Creator/1  "Vb"

== system test_bu01_2018b_tuning/Plant/bu01_model/动力系统模型/Motor7_PF_N/PFKV2300 ==
  Um : Inport  PortDimensions=1
  Tq : Inport  Port=2  PortDimensions=1
  Izz : Inport  Port=3  PortDimensions=1
  Bus Selector : BusSelector  OutputSignals=Im,RPM
  Bus Creator : BusCreator  Inputs=3
  DCMotor : Subsystem  mask{L=0.0053, Km=0.0041, Kemf=0.0041, Imzz=1e-05, Ra=0.045, I0=2.35}
      mask prompts: L "电感值L"; Km "转矩常量Km"; Kemf "反电动势Kemf"; Imzz "转子惯量Imzz"; Ra "电动机内阻Ra"; I0 "空载电流I0"
      mask Display: disp('DCMotor')
  Im : Outport
  RPM : Outport  Port=2
  wires:
  Bus Creator/1 -> DCMotor/1(In1)
  Um/1 -> Bus Creator/1  "Um"
  Izz/1 -> Bus Creator/3  "Izz"
  Bus Selector/2 -> RPM/1  "<RPM>"
  Tq/1 -> Bus Creator/2  "Tq"
  DCMotor/1(Out1) -> Bus Selector/1
  Bus Selector/1 -> Im/1  "<Im>"

== system test_bu01_2018b_tuning/Plant/bu01_model/动力系统模型/Motor8_PF_N/PF70mmDuctFanN ==
  Vb_ip : Inport  PortDimensions=3
  Wb_ip : Inport  Port=2  PortDimensions=3
  Ax_ip : Inport  Port=3  PortDimensions=3
  Ns_ip : Inport  Port=4  PortDimensions=1
  Pro : Inport  Port=5  PortDimensions=1
  Bus Selector : BusSelector  OutputSignals=Fb&Mb,Tq,Izz
  Bus Selector1 : BusSelector  OutputSignals=Fb,Mb
  Bus Creator : BusCreator  Inputs=5
  "涵道风扇模型 " : Subsystem  mask{Fratio=1.125, Mratio=0.975, Tqratio=0.4, Izz=0.00000309}
      mask prompts: Fratio "涵道风扇气动力修正系数"; Mratio "涵道风扇气动力矩修正系数"; Tqratio "涵道风扇扭矩修正系数"; Izz "涵道风扇转动惯量"
  Fb : Outport
  Mb : Outport  Port=2
  Tq : Outport  Port=3
  Izz : Outport  Port=4
  wires:
  Vb_ip/1 -> Bus Creator/1  "Vb"
  Ax_ip/1 -> Bus Creator/3  "Ax"
  "涵道风扇模型 "/1(Out1) -> Bus Selector/1
  Bus Creator/1 -> "涵道风扇模型 "/1(In1)
  Wb_ip/1 -> Bus Creator/2  "Wb"
  Bus Selector/1 -> Bus Selector1/1  "<Fb&Mb>"
  Bus Selector1/2 -> Mb/1  "<Mb>"
  Ns_ip/1 -> Bus Creator/4  "Ns"
  Bus Selector1/1 -> Fb/1  "<Fb>"
  Bus Selector/3 -> Izz/1  "<Izz>"
  Bus Selector/2 -> Tq/1  "<Tq>"
  Pro/1 -> Bus Creator/5  "Pro"

== system test_bu01_2018b_tuning/Plant/bu01_model/动力系统模型/Motor8_PF_N/PFKV2300 ==
  Um : Inport  PortDimensions=1
  Tq : Inport  Port=2  PortDimensions=1
  Izz : Inport  Port=3  PortDimensions=1
  Bus Selector : BusSelector  OutputSignals=Im,RPM
  Bus Creator : BusCreator  Inputs=3
  DCMotor : Subsystem  mask{L=0.0053, Km=0.0041, Kemf=0.0041, Imzz=1e-05, Ra=0.045, I0=2.35}
      mask prompts: L "电感值L"; Km "转矩常量Km"; Kemf "反电动势Kemf"; Imzz "转子惯量Imzz"; Ra "电动机内阻Ra"; I0 "空载电流I0"
      mask Display: disp('DCMotor')
  Im : Outport
  RPM : Outport  Port=2
  wires:
  Bus Selector/1 -> Im/1  "<Im>"
  DCMotor/1(Out1) -> Bus Selector/1
  Tq/1 -> Bus Creator/2  "Tq"
  Bus Selector/2 -> RPM/1  "<RPM>"
  Izz/1 -> Bus Creator/3  "Izz"
  Um/1 -> Bus Creator/1  "Um"
  Bus Creator/1 -> DCMotor/1(In1)

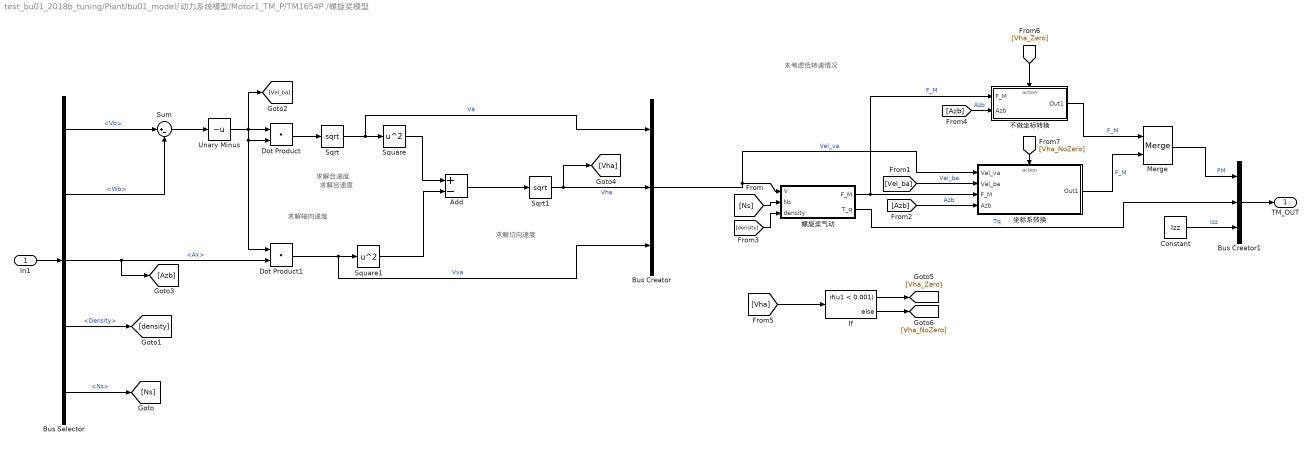
== system test_bu01_2018b_tuning/Plant/bu01_model/动力系统模型/Motor1_TM_P/TM1654P /螺旋桨模型 ==
  note: 未考虑低转速情况
  note: 求解合速度
  note: 求解轴向速度
  note: 求解切向速度
  note: 求解合速度
  In1 : Inport
  Add : Sum  Inputs=+-
  Bus Selector : BusSelector  OutputSignals=Vb,Wb,Ax,Density,Ns
  Bus Creator : BusCreator  Inputs=3
  Bus Creator1 : BusCreator  Inputs=3
  Constant : Constant  Value=Izz  OutDataTypeStr=double
  Dot Product : DotProduct  InputSameDT=on  OutDataTypeStr=Inherit: Inherit via internal rule
  Dot Product1 : DotProduct  InputSameDT=on  OutDataTypeStr=Inherit: Inherit via internal rule
  If : If  IfExpression=u1 < 0.001
  Merge : Merge
  Sqrt : Sqrt  SaturateOnIntegerOverflow=on
  Sqrt1 : Sqrt  SaturateOnIntegerOverflow=on
  Square : Math  Operator=square  SaturateOnIntegerOverflow=on
  Square1 : Math  Operator=square  SaturateOnIntegerOverflow=on
  Sum : Sum  Inputs=|+-
  Unary Minus : UnaryMinus
  不做坐标转换 : Subsystem
  坐标系转换 : Subsystem
  螺旋桨气动 : Subsystem
  TM_OUT : Outport
  wires:
  In1/1 -> Bus Selector/1
  Bus Selector/1 -> Sum/1  "<Vb>"
  Bus Selector/2 -> Sum/2  "<Wb>"
  Sum/1 -> Unary Minus/1
  Unary Minus/1 -> [Vel_ba], Dot Product/2, Dot Product1/1, Dot Product/1
  Dot Product/1 -> Sqrt/1
  Sqrt/1 -> Bus Creator/1, Square/1  "Va"
  Bus Selector/3 -> [Azb], Dot Product1/2  "<Ax>"
  Bus Selector/4 -> [density]  "<Density>"
  Bus Selector/5 -> [Ns]  "<Ns>"
  Dot Product1/1 -> Bus Creator/3, Square1/1  "Vva"
  Square1/1 -> Add/2
  Square/1 -> Add/1
  Add/1 -> Sqrt1/1
  Sqrt1/1 -> [Vha], Bus Creator/2  "Vha"
  Bus Creator/1 -> 坐标系转换/1(Vel_va), 螺旋桨气动/1(V)  "Vel_va"
  [Ns] -> 螺旋桨气动/2(Ns)
  [Vel_ba] -> 坐标系转换/2(Vel_ba)  "Vel_ba"
  螺旋桨气动/1(F_M) -> 不做坐标转换/1(F_M), 坐标系转换/3(F_M)  "F_M"
  [Azb] -> 坐标系转换/4(Azb)  "Azb"
  [density] -> 螺旋桨气动/3(density)
  螺旋桨气动/2(T_q) -> Bus Creator1/2  "Tq"
  Constant/1 -> Bus Creator1/3  "Izz"
  Bus Creator1/1 -> TM_OUT/1
  [Azb] -> 不做坐标转换/2(Azb)  "Azb"
  [Vha] -> If/1
  不做坐标转换/1(Out1) -> Merge/1  "F_M"
  坐标系转换/1(Out1) -> Merge/2  "F_M"
  Merge/1 -> Bus Creator1/1  "FM"
  If/1 -> [Vha_Zero]
  If/2 -> [Vha_NoZero]
  [Vha_Zero] -> 不做坐标转换/Action
  [Vha_NoZero] -> 坐标系转换/Action

== system test_bu01_2018b_tuning/Plant/bu01_model/动力系统模型/Motor1_TM_P/TMU5KV400 /DCMotor ==
  In1 : Inport
  Add : Sum  Inputs=+--
  Add1 : Sum  Inputs=+-
  Add2 : Sum
  Add3 : Sum  Inputs=+-
  Bus Selector : BusSelector  OutputSignals=Um,Tq,Izz
  Bus Creator : BusCreator  Inputs=2
  Constant : Constant  Value=Imzz
  Constant1 : Constant  Value=I0
  Divide : Product  Inputs=*/
  Gain : Gain  Gain=1/L
  Gain1 : Gain  Gain=Km
  Gain3 : Gain  Gain=Kemf
  Gain4 : Gain  Gain=Ra
  Gain5 : Gain  Gain=1/(2*pi)
  Gain6 : Gain  Gain=60
  Integrator : Integrator  InitialCondition=0.0001
  Integrator1 : Integrator  InitialCondition=0.0001
  Multiply : Product
  Multiply1 : Product
  Terminator : Terminator
  Terminator1 : Terminator
  Out1 : Outport
  wires:
  In1/1 -> Bus Selector/1
  Bus Selector/1 -> Multiply/1, Add/1  "<Um>"
  Add/1 -> Gain/1
  Gain/1 -> Integrator/1
  Integrator/1 -> Add3/1, Multiply/2, Bus Creator/1, Gain4/1  "Im"
  Gain1/1 -> Multiply1/1, Add1/1  "Te"
  Integrator1/1 -> Multiply1/2, Gain3/1, Gain5/1  "w"
  Add1/1 -> Divide/1
  Divide/1 -> Integrator1/1
  Gain3/1 -> Add/2  "Ea"
  Gain4/1 -> Add/3
  Bus Selector/2 -> [Tq]  "<Tq>"
  Bus Selector/3 -> Add2/1  "<Izz>"
  Constant/1 -> Add2/2
  Add2/1 -> [J]
  [J] -> Divide/2
  Multiply/1 -> Terminator/1  "Pwin"
  Multiply1/1 -> Terminator1/1  "Pwout"
  Gain5/1 -> Gain6/1  "RPS"
  Gain6/1 -> Bus Creator/2  "RPM"
  Bus Creator/1 -> Out1/1
  [Tq] -> Add1/2
  Add3/1 -> Gain1/1  "Iav"
  Constant1/1 -> Add3/2

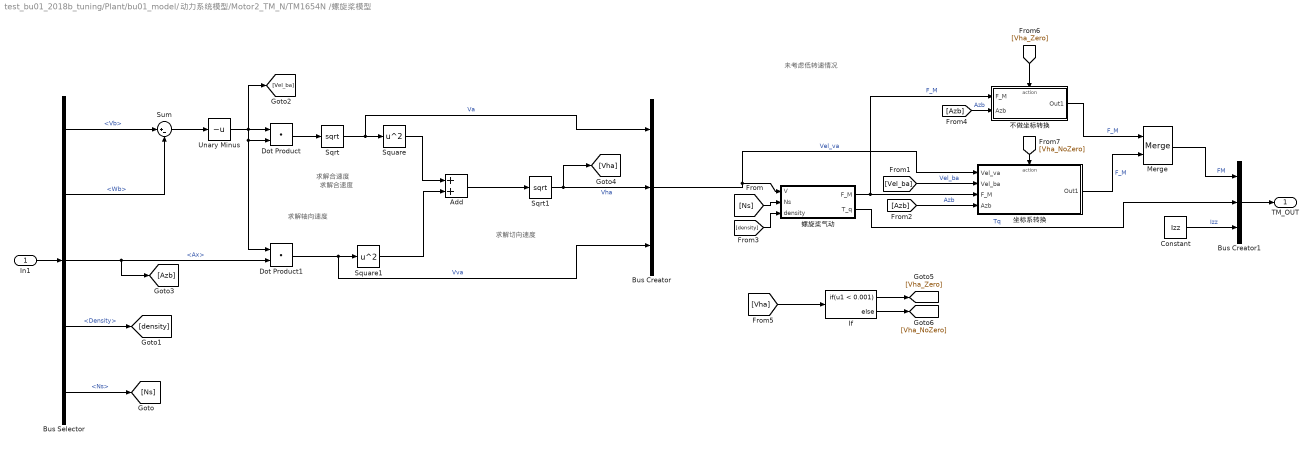
== system test_bu01_2018b_tuning/Plant/bu01_model/动力系统模型/Motor2_TM_N/TM1654N /螺旋桨模型 ==
  note: 未考虑低转速情况
  note: 求解合速度
  note: 求解轴向速度
  note: 求解切向速度
  note: 求解合速度
  In1 : Inport
  Add : Sum
  Bus Selector : BusSelector  OutputSignals=Vb,Wb,Ax,Density,Ns
  Bus Creator : BusCreator  Inputs=3
  Bus Creator1 : BusCreator  Inputs=3
  Constant : Constant  Value=Izz  OutDataTypeStr=double
  Dot Product : DotProduct  InputSameDT=on  OutDataTypeStr=Inherit: Inherit via internal rule
  Dot Product1 : DotProduct  InputSameDT=on  OutDataTypeStr=Inherit: Inherit via internal rule
  If : If  IfExpression=u1 < 0.001
  Merge : Merge
  Sqrt : Sqrt  SaturateOnIntegerOverflow=on
  Sqrt1 : Sqrt  SaturateOnIntegerOverflow=on
  Square : Math  Operator=square  SaturateOnIntegerOverflow=on
  Square1 : Math  Operator=square  SaturateOnIntegerOverflow=on
  Sum : Sum  Inputs=|+-
  Unary Minus : UnaryMinus
  不做坐标转换 : Subsystem
  坐标系转换 : Subsystem
  螺旋桨气动 : Subsystem
  TM_OUT : Outport
  wires:
  In1/1 -> Bus Selector/1
  Bus Selector/1 -> Sum/1  "<Vb>"
  Bus Selector/2 -> Sum/2  "<Wb>"
  Sum/1 -> Unary Minus/1
  Unary Minus/1 -> [Vel_ba], Dot Product/2, Dot Product1/1, Dot Product/1
  Dot Product/1 -> Sqrt/1
  Sqrt/1 -> Bus Creator/1, Square/1  "Va"
  Bus Selector/3 -> [Azb], Dot Product1/2  "<Ax>"
  Bus Selector/4 -> [density]  "<Density>"
  Bus Selector/5 -> [Ns]  "<Ns>"
  Dot Product1/1 -> Bus Creator/3, Square1/1  "Vva"
  Square1/1 -> Add/2
  Square/1 -> Add/1
  Add/1 -> Sqrt1/1
  Sqrt1/1 -> [Vha], Bus Creator/2  "Vha"
  Bus Creator/1 -> 坐标系转换/1(Vel_va), 螺旋桨气动/1(V)  "Vel_va"
  [Ns] -> 螺旋桨气动/2(Ns)
  [Vel_ba] -> 坐标系转换/2(Vel_ba)  "Vel_ba"
  螺旋桨气动/1(F_M) -> 不做坐标转换/1(F_M), 坐标系转换/3(F_M)  "F_M"
  [Azb] -> 坐标系转换/4(Azb)  "Azb"
  [density] -> 螺旋桨气动/3(density)
  螺旋桨气动/2(T_q) -> Bus Creator1/2  "Tq"
  Constant/1 -> Bus Creator1/3  "Izz"
  Bus Creator1/1 -> TM_OUT/1
  [Azb] -> 不做坐标转换/2(Azb)  "Azb"
  [Vha] -> If/1
  不做坐标转换/1(Out1) -> Merge/1  "F_M"
  坐标系转换/1(Out1) -> Merge/2  "F_M"
  Merge/1 -> Bus Creator1/1  "FM"
  If/1 -> [Vha_Zero]
  If/2 -> [Vha_NoZero]
  [Vha_Zero] -> 不做坐标转换/Action
  [Vha_NoZero] -> 坐标系转换/Action

== system test_bu01_2018b_tuning/Plant/bu01_model/动力系统模型/Motor2_TM_N/TMU5KV400 /DCMotor1 ==
  In1 : Inport
  Add : Sum  Inputs=+--
  Add1 : Sum  Inputs=+-
  Add2 : Sum
  Add3 : Sum  Inputs=+-
  Bus Selector : BusSelector  OutputSignals=Um,Tq,Izz
  Bus Creator : BusCreator  Inputs=2
  Constant : Constant  Value=Imzz
  Constant1 : Constant  Value=I0
  Divide : Product  Inputs=*/
  Gain : Gain  Gain=1/L
  Gain1 : Gain  Gain=Km
  Gain3 : Gain  Gain=Kemf
  Gain4 : Gain  Gain=Ra
  Gain5 : Gain  Gain=1/(2*pi)
  Gain6 : Gain  Gain=60
  Integrator : Integrator  InitialCondition=0.0001
  Integrator1 : Integrator  InitialCondition=0.0001
  Multiply : Product
  Multiply1 : Product
  Terminator : Terminator
  Terminator1 : Terminator
  Out1 : Outport
  wires:
  In1/1 -> Bus Selector/1
  Bus Selector/1 -> Multiply/1, Add/1  "<Um>"
  Add/1 -> Gain/1
  Gain/1 -> Integrator/1
  Integrator/1 -> Add3/1, Multiply/2, Bus Creator/1, Gain4/1  "Im"
  Gain1/1 -> Multiply1/1, Add1/1  "Te"
  Integrator1/1 -> Multiply1/2, Gain3/1, Gain5/1  "w"
  Add1/1 -> Divide/1
  Divide/1 -> Integrator1/1
  Gain3/1 -> Add/2  "Ea"
  Gain4/1 -> Add/3
  Bus Selector/2 -> [Tq]  "<Tq>"
  Bus Selector/3 -> Add2/1  "<Izz>"
  Constant/1 -> Add2/2
  Add2/1 -> [J]
  [J] -> Divide/2
  Multiply/1 -> Terminator/1  "Pwin"
  Multiply1/1 -> Terminator1/1  "Pwout"
  Gain5/1 -> Gain6/1  "RPS"
  Gain6/1 -> Bus Creator/2  "RPM"
  Bus Creator/1 -> Out1/1
  [Tq] -> Add1/2
  Add3/1 -> Gain1/1  "Iav"
  Constant1/1 -> Add3/2

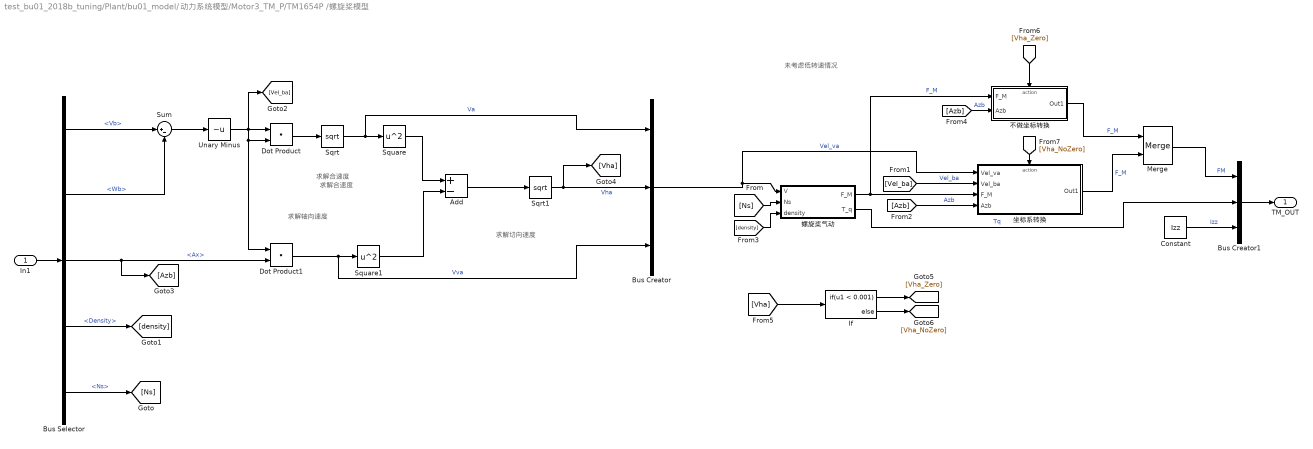
== system test_bu01_2018b_tuning/Plant/bu01_model/动力系统模型/Motor3_TM_P/TM1654P /螺旋桨模型 ==
  note: 未考虑低转速情况
  note: 求解合速度
  note: 求解轴向速度
  note: 求解切向速度
  note: 求解合速度
  In1 : Inport
  Add : Sum  Inputs=+-
  Bus Selector : BusSelector  OutputSignals=Vb,Wb,Ax,Density,Ns
  Bus Creator : BusCreator  Inputs=3
  Bus Creator1 : BusCreator  Inputs=3
  Constant : Constant  Value=Izz  OutDataTypeStr=double
  Dot Product : DotProduct  InputSameDT=on  OutDataTypeStr=Inherit: Inherit via internal rule
  Dot Product1 : DotProduct  InputSameDT=on  OutDataTypeStr=Inherit: Inherit via internal rule
  If : If  IfExpression=u1 < 0.001
  Merge : Merge
  Sqrt : Sqrt  SaturateOnIntegerOverflow=on
  Sqrt1 : Sqrt  SaturateOnIntegerOverflow=on
  Square : Math  Operator=square  SaturateOnIntegerOverflow=on
  Square1 : Math  Operator=square  SaturateOnIntegerOverflow=on
  Sum : Sum  Inputs=|+-
  Unary Minus : UnaryMinus
  不做坐标转换 : Subsystem
  坐标系转换 : Subsystem
  螺旋桨气动 : Subsystem
  TM_OUT : Outport
  wires:
  In1/1 -> Bus Selector/1
  Bus Selector/1 -> Sum/1  "<Vb>"
  Bus Selector/2 -> Sum/2  "<Wb>"
  Sum/1 -> Unary Minus/1
  Unary Minus/1 -> [Vel_ba], Dot Product/2, Dot Product1/1, Dot Product/1
  Dot Product/1 -> Sqrt/1
  Sqrt/1 -> Bus Creator/1, Square/1  "Va"
  Bus Selector/3 -> [Azb], Dot Product1/2  "<Ax>"
  Bus Selector/4 -> [density]  "<Density>"
  Bus Selector/5 -> [Ns]  "<Ns>"
  Dot Product1/1 -> Bus Creator/3, Square1/1  "Vva"
  Square1/1 -> Add/2
  Square/1 -> Add/1
  Add/1 -> Sqrt1/1
  Sqrt1/1 -> [Vha], Bus Creator/2  "Vha"
  Bus Creator/1 -> 坐标系转换/1(Vel_va), 螺旋桨气动/1(V)  "Vel_va"
  [Ns] -> 螺旋桨气动/2(Ns)
  [Vel_ba] -> 坐标系转换/2(Vel_ba)  "Vel_ba"
  螺旋桨气动/1(F_M) -> 不做坐标转换/1(F_M), 坐标系转换/3(F_M)  "F_M"
  [Azb] -> 坐标系转换/4(Azb)  "Azb"
  [density] -> 螺旋桨气动/3(density)
  螺旋桨气动/2(T_q) -> Bus Creator1/2  "Tq"
  Constant/1 -> Bus Creator1/3  "Izz"
  Bus Creator1/1 -> TM_OUT/1
  [Azb] -> 不做坐标转换/2(Azb)  "Azb"
  [Vha] -> If/1
  不做坐标转换/1(Out1) -> Merge/1  "F_M"
  坐标系转换/1(Out1) -> Merge/2  "F_M"
  Merge/1 -> Bus Creator1/1  "FM"
  If/1 -> [Vha_Zero]
  If/2 -> [Vha_NoZero]
  [Vha_Zero] -> 不做坐标转换/Action
  [Vha_NoZero] -> 坐标系转换/Action

== system test_bu01_2018b_tuning/Plant/bu01_model/动力系统模型/Motor3_TM_P/TMU5KV400 /DCMotor ==
  In1 : Inport
  Add : Sum  Inputs=+--
  Add1 : Sum  Inputs=+-
  Add2 : Sum
  Add3 : Sum  Inputs=+-
  Bus Selector : BusSelector  OutputSignals=Um,Tq,Izz
  Bus Creator : BusCreator  Inputs=2
  Constant : Constant  Value=Imzz
  Constant1 : Constant  Value=I0
  Divide : Product  Inputs=*/
  Gain : Gain  Gain=1/L
  Gain1 : Gain  Gain=Km
  Gain3 : Gain  Gain=Kemf
  Gain4 : Gain  Gain=Ra
  Gain5 : Gain  Gain=1/(2*pi)
  Gain6 : Gain  Gain=60
  Integrator : Integrator  InitialCondition=0.0001
  Integrator1 : Integrator  InitialCondition=0.0001
  Multiply : Product
  Multiply1 : Product
  Terminator : Terminator
  Terminator1 : Terminator
  Out1 : Outport
  wires:
  In1/1 -> Bus Selector/1
  Bus Selector/1 -> Multiply/1, Add/1  "<Um>"
  Add/1 -> Gain/1
  Gain/1 -> Integrator/1
  Integrator/1 -> Add3/1, Multiply/2, Bus Creator/1, Gain4/1  "Im"
  Gain1/1 -> Multiply1/1, Add1/1  "Te"
  Integrator1/1 -> Multiply1/2, Gain3/1, Gain5/1  "w"
  Add1/1 -> Divide/1
  Divide/1 -> Integrator1/1
  Gain3/1 -> Add/2  "Ea"
  Gain4/1 -> Add/3
  Bus Selector/2 -> [Tq]  "<Tq>"
  Bus Selector/3 -> Add2/1  "<Izz>"
  Constant/1 -> Add2/2
  Add2/1 -> [J]
  [J] -> Divide/2
  Multiply/1 -> Terminator/1  "Pwin"
  Multiply1/1 -> Terminator1/1  "Pwout"
  Gain5/1 -> Gain6/1  "RPS"
  Gain6/1 -> Bus Creator/2  "RPM"
  Bus Creator/1 -> Out1/1
  [Tq] -> Add1/2
  Add3/1 -> Gain1/1  "Iav"
  Constant1/1 -> Add3/2

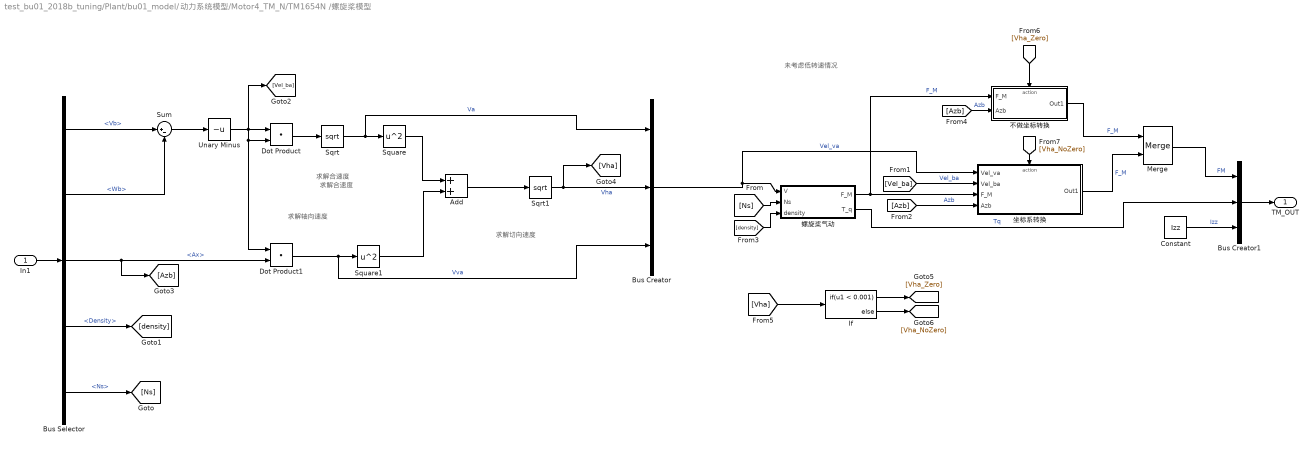
== system test_bu01_2018b_tuning/Plant/bu01_model/动力系统模型/Motor4_TM_N/TM1654N /螺旋桨模型 ==
  note: 未考虑低转速情况
  note: 求解合速度
  note: 求解轴向速度
  note: 求解切向速度
  note: 求解合速度
  In1 : Inport
  Add : Sum
  Bus Selector : BusSelector  OutputSignals=Vb,Wb,Ax,Density,Ns
  Bus Creator : BusCreator  Inputs=3
  Bus Creator1 : BusCreator  Inputs=3
  Constant : Constant  Value=Izz  OutDataTypeStr=double
  Dot Product : DotProduct  InputSameDT=on  OutDataTypeStr=Inherit: Inherit via internal rule
  Dot Product1 : DotProduct  InputSameDT=on  OutDataTypeStr=Inherit: Inherit via internal rule
  If : If  IfExpression=u1 < 0.001
  Merge : Merge
  Sqrt : Sqrt  SaturateOnIntegerOverflow=on
  Sqrt1 : Sqrt  SaturateOnIntegerOverflow=on
  Square : Math  Operator=square  SaturateOnIntegerOverflow=on
  Square1 : Math  Operator=square  SaturateOnIntegerOverflow=on
  Sum : Sum  Inputs=|+-
  Unary Minus : UnaryMinus
  不做坐标转换 : Subsystem
  坐标系转换 : Subsystem
  螺旋桨气动 : Subsystem
  TM_OUT : Outport
  wires:
  In1/1 -> Bus Selector/1
  Bus Selector/1 -> Sum/1  "<Vb>"
  Bus Selector/2 -> Sum/2  "<Wb>"
  Sum/1 -> Unary Minus/1
  Unary Minus/1 -> [Vel_ba], Dot Product/2, Dot Product1/1, Dot Product/1
  Dot Product/1 -> Sqrt/1
  Sqrt/1 -> Bus Creator/1, Square/1  "Va"
  Bus Selector/3 -> [Azb], Dot Product1/2  "<Ax>"
  Bus Selector/4 -> [density]  "<Density>"
  Bus Selector/5 -> [Ns]  "<Ns>"
  Dot Product1/1 -> Bus Creator/3, Square1/1  "Vva"
  Square1/1 -> Add/2
  Square/1 -> Add/1
  Add/1 -> Sqrt1/1
  Sqrt1/1 -> [Vha], Bus Creator/2  "Vha"
  Bus Creator/1 -> 坐标系转换/1(Vel_va), 螺旋桨气动/1(V)  "Vel_va"
  [Ns] -> 螺旋桨气动/2(Ns)
  [Vel_ba] -> 坐标系转换/2(Vel_ba)  "Vel_ba"
  螺旋桨气动/1(F_M) -> 不做坐标转换/1(F_M), 坐标系转换/3(F_M)  "F_M"
  [Azb] -> 坐标系转换/4(Azb)  "Azb"
  [density] -> 螺旋桨气动/3(density)
  螺旋桨气动/2(T_q) -> Bus Creator1/2  "Tq"
  Constant/1 -> Bus Creator1/3  "Izz"
  Bus Creator1/1 -> TM_OUT/1
  [Azb] -> 不做坐标转换/2(Azb)  "Azb"
  [Vha] -> If/1
  不做坐标转换/1(Out1) -> Merge/1  "F_M"
  坐标系转换/1(Out1) -> Merge/2  "F_M"
  Merge/1 -> Bus Creator1/1  "FM"
  If/1 -> [Vha_Zero]
  If/2 -> [Vha_NoZero]
  [Vha_Zero] -> 不做坐标转换/Action
  [Vha_NoZero] -> 坐标系转换/Action
